simulink model "test2"  (R2016a)
settings: Solver=VariableStepAuto  StartTime=0.0  StopTime=10.0  RelTol=1e-3
values from neighbouring files (symbols this model uses):
  BitRate = 10000    [test2m1.m]    (also in test2m2.m)
  K = 4    [test2m1.m]    (also in test2m2.m = 26)
  x = -10:1:10    [test2m1.m]    (also in test2m2.m)
undefined symbols (not defined in the file or in its folder): i
libraries: commdigbbndpm3 x2, commblkcod2 x2, commchan3 x1, commsink2 x1, commrandsrc3 x1
settings Model: Creator=Han Solo  LastModifiedBy=Han Solo

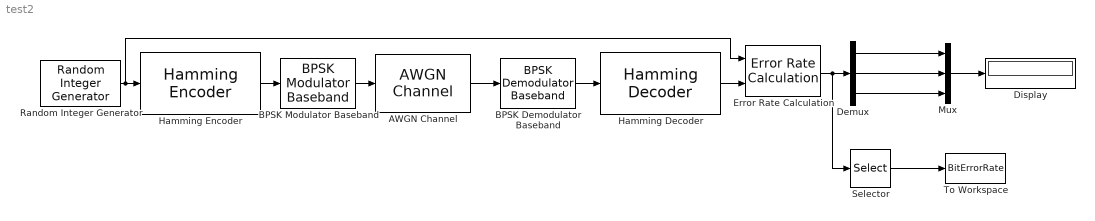
== system test2 ==
  AWGN Channel : commchan3/AWGN Channel  InputProcessing=Columns as channels (frame based)  seed=67  noiseMode="Signal to noise ratio  (SNR)"  EbNodB=10  EsNodB=10  SNRdB=x(i)  bitsPerSym=1  Ps=1  Tsym=1  variance=1
  BPSK Demodulator Baseband : commdigbbndpm3/BPSK Demodulator Baseband  DecType=Hard decision  VarSource=Dialog  Variance=1  Ph=pi/8  outDtype=Inherit via internal rule  derotateFactorWordLen=16  derotateFactorDataTypeStr=Inherit: Same word length as input  derotateFactorLastDataTypeStr=Inherit: Same word length as input
  BPSK Modulator Baseband : commdigbbndpm3/BPSK Modulator Baseband  Ph=pi/8  outDtype=double  outWordLen=16  outUDDataType=sfix(16)  outFracLenMode=Best precision  outFracLen=15  outDataTypeStr=double  outLastDataTypeStr=double
  Demux : Demux  Outputs=3
  Display : Display
  Error Rate Calculation : commsink2/Error Rate Calculation  N=0  st_delay=0  cp_mode=Entire frame  subframe=[]  PMode=Port  WsName=ErrorVec  RsMode2=off  stop=off  numErr=100  maxBits=1e6
  Hamming Decoder : commblkcod2/Hamming Decoder  n=N  k=K
  Hamming Encoder : commblkcod2/Hamming Encoder  n=N  k=K
  Mux : Mux  Inputs=3
  Random Integer Generator : commrandsrc3/Random Integer Generator  SetSize=2  SeedSource=Parameter  Seed=37  SampleTime=1/BitRate  SamplesPerFrame=S  OutputDataType=double  SimulateUsing=Interpreted execution
  Selector : Selector  InputPortWidth=3  IndexOptions=Index vector (dialog)  Indices=[1]  OutputSizes=1
  To Workspace : ToWorkspace  VariableName=BitErrorRate  SampleTime=-1
  wires:
  BPSK Modulator Baseband/1 -> AWGN Channel/1
  Hamming Encoder/1 -> BPSK Modulator Baseband/1
  Mux/1 -> Display/1
  BPSK Demodulator Baseband/1 -> Hamming Decoder/1
  Hamming Decoder/1 -> Error Rate Calculation/2
  Random Integer Generator/1 -> Error Rate Calculation/1, Hamming Encoder/1
  Error Rate Calculation/1 -> Selector/1, Demux/1
  Selector/1 -> To Workspace/1
  Demux/1 -> Mux/1
  Demux/2 -> Mux/2
  Demux/3 -> Mux/3
  AWGN Channel/1 -> BPSK Demodulator Baseband/1
